simulink model "es3"  (R2022b)
settings: Solver=VariableStepAuto  StartTime=0.0  StopTime=2  RelTol=1e-3
settings Model: Creator=adlercohen  LastModifiedBy=adlercohen

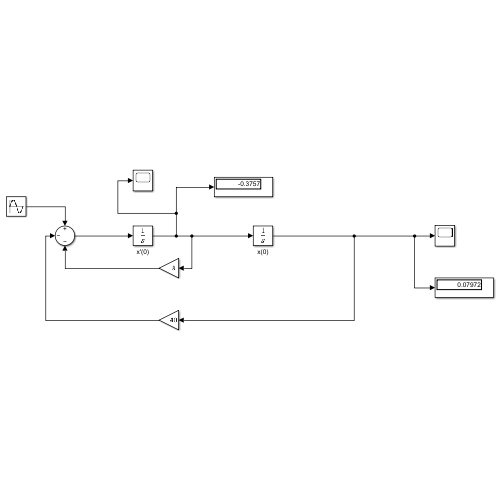
[thumbnail: Simulink's stored preview of the top-level diagram]
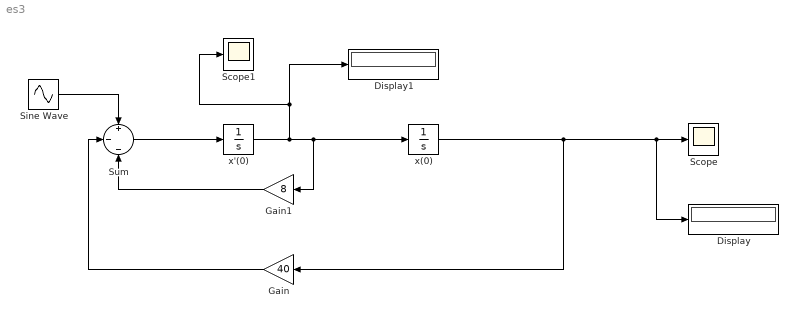
== system es3 ==
  Display : Display
  Display1 : Display
  Gain : Gain  Gain=40
  Gain1 : Gain  Gain=8
  Scope : Scope
  Scope1 : Scope
  Sine Wave : Sin  Amplitude=10  Frequency=pi/2  SampleTime=0
  Sum : Sum  Inputs=+|-|-
  x'(0) : Integrator  InitialCondition=2.5
  x(0) : Integrator  InitialCondition=1
  wires:
  x'(0)/1 -> Display1/1, Scope1/1, Gain1/1, x(0)/1
  Sum/1 -> x'(0)/1
  Gain/1 -> Sum/2
  Gain1/1 -> Sum/3
  x(0)/1 -> Scope/1, Display/1, Gain/1
  Sine Wave/1 -> Sum/1
